simulink model "Lab2_PartA1"  (R2025b)
settings: Solver=VariableStepAuto  StartTime=0.0  StopTime=10.0  RelTol=1e-3
libraries: SignalEditorBlockLib x1
settings Model: Creator=Murl0  LastModifiedBy=Murl0

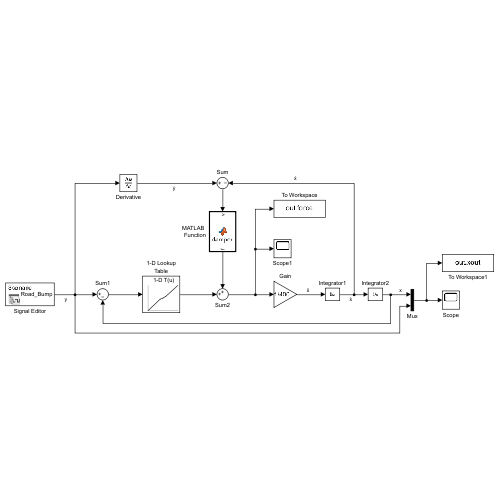
[thumbnail: Simulink's stored preview of the top-level diagram]
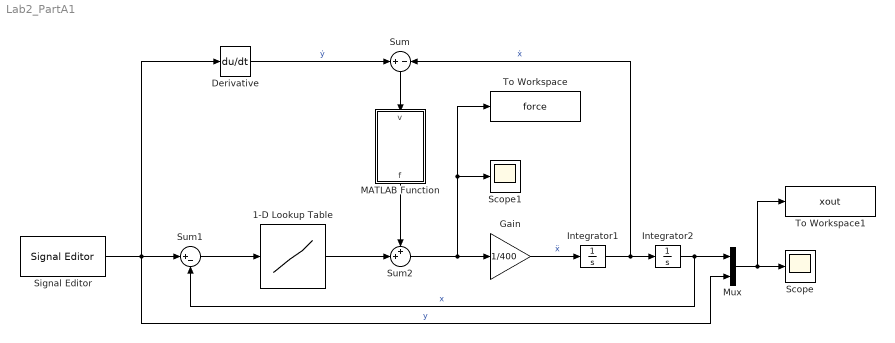
== system Lab2_PartA1 ==
  1-D Lookup Table : Lookup_n-D  NumberOfTableDimensions=1  BreakpointsForDimension1=[-0.5;-0.1;0;0.1;0.5]  Table=[-4500;-500;0;500;4500]  InternalRulePriority=Speed  RndMeth=Simplest
  Derivative : Derivative
  Gain : Gain  Gain=1/400
  Integrator1 : Integrator
  Integrator2 : Integrator
  MATLAB Function : MATLAB Function  TreatAsAtomicUnit=on
  Mux : Mux  Inputs=2
  Scope : Scope
      settings: ActiveDisplayYMinimum=-0.2175099484965356  ActiveDisplayYMaximum=0.310641951430441
  Scope1 : Scope
      settings: ActiveDisplayYMinimum=-2740.6779701836936  ActiveDisplayYMaximum=2179.1010694395995
  Signal Editor : SignalEditorBlockLib/Signal Editor  FileName=Input.mat  ActiveScenario=Scenario  ActiveSignal=Road_Bump  IsBus=off  OutputBusObjectStr=Bus: BusObject  SampleTime=0  ZeroCross=off  OutputAfterFinalValue=Setting to zero  Unit=m  PreserveSignalName=on  ApplySigPropsToAllScenarios=on  ApplySigPropsToAllSignals=off  SignalPropertySource=Dialog parameters
  Sum : Sum  Inputs=+-
  Sum1 : Sum  Inputs=|+-
  Sum2 : Sum  Inputs=++|
  To Workspace : ToWorkspace  VariableName=force  SampleTime=-1
  To Workspace1 : ToWorkspace  VariableName=xout  SampleTime=-1
  wires:
  Mux/1 -> Scope/1, To Workspace1/1
  Integrator2/1 -> Mux/1, Sum1/2  "x"
  Integrator1/1 -> Sum/2, Integrator2/1  "ẋ"
  Gain/1 -> Integrator1/1  "ẍ"
  Sum2/1 -> Gain/1, Scope1/1, To Workspace/1
  MATLAB Function/1(f) -> Sum2/1
  Sum/1 -> MATLAB Function/1(v)
  Derivative/1 -> Sum/1  "ẏ"
  1-D Lookup Table/1 -> Sum2/2
  Sum1/1 -> 1-D Lookup Table/1
  Signal Editor/1 -> Derivative/1, Sum1/1, Mux/2  "y"

== matlab function Lab2_PartA1/MATLAB Function ==
  data: v input; f output
function f = damper(v)

if v<= 0
    f = -800*(abs(v)).^(0.6);
else
    f = 200*v.^(0.6);
end
